simulink model "SimulacionDataRealLaptop"  (R2022b)
settings: Solver=ode4  StartTime=0.0  StopTime=60  FixedStep=0.001  RelTol=1e-3
undefined symbols (not defined in the file): k1, k2, nq, P, W1_0, W2_0
settings Model: Creator=raul  LastModifiedBy=raul

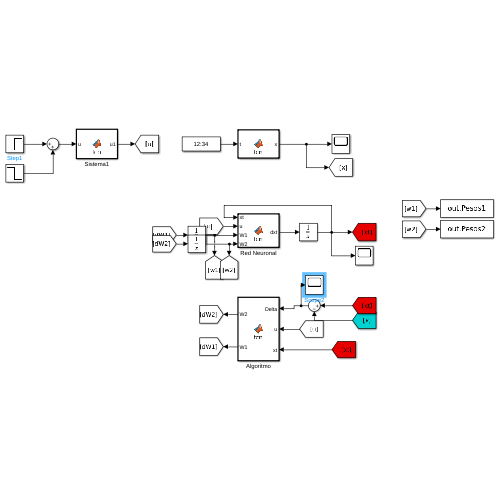
[thumbnail: Simulink's stored preview of the top-level diagram]
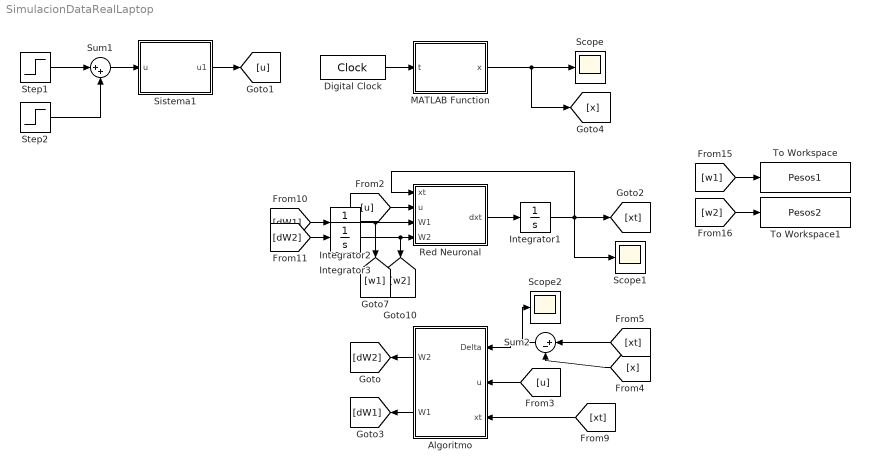
== system SimulacionDataRealLaptop ==
  Algoritmo : MATLAB Function  TreatAsAtomicUnit=on
  Digital Clock : DigitalClock  SampleTime=0.01
  Integrator1 : Integrator  InitialCondition=zeros(2*nq,1)
  Integrator2 : Integrator  InitialCondition=W1_0
  Integrator3 : Integrator  InitialCondition=W2_0
  MATLAB Function : MATLAB Function  TreatAsAtomicUnit=on
  Red Neuronal : MATLAB Function  TreatAsAtomicUnit=on
  Scope : Scope
  Scope1 : Scope
  Scope2 : Scope
  Sistema1 : MATLAB Function  TreatAsAtomicUnit=on
  Step1 : Step  Time=13.50  After=15  SampleTime=0
  Step2 : Step  Time=14  After=-15  SampleTime=0
  Sum1 : Sum  Inputs=|++
  Sum2 : Sum  Inputs=|+-
  To Workspace : ToWorkspace  VariableName=Pesos1  SampleTime=-1
  To Workspace1 : ToWorkspace  VariableName=Pesos2  SampleTime=-1
  wires:
  Digital Clock/1 -> MATLAB Function/1(t)
  MATLAB Function/1(x) -> [x], Scope/1
  [x] -> Sum2/2
  [dW2] -> Integrator3/1
  Integrator3/1 -> [w2], Red Neuronal/4(W2)
  [xt] -> Algoritmo/3(xt)
  Algoritmo/2(W1) -> [dW1]
  Algoritmo/1(W2) -> [dW2]
  [u] -> Algoritmo/2(u)
  [u] -> Red Neuronal/2(u)
  Integrator1/1 -> Scope1/1, [xt], Red Neuronal/1(xt)
  Red Neuronal/1(dxt) -> Integrator1/1
  [xt] -> Sum2/1
  Integrator2/1 -> [w1], Red Neuronal/3(W1)
  [dW1] -> Integrator2/1
  Sum2/1 -> Scope2/1, Algoritmo/1(Delta)
  [w2] -> To Workspace1/1
  [w1] -> To Workspace/1
  Step1/1 -> Sum1/1
  Sum1/1 -> Sistema1/1(u)
  Step2/1 -> Sum1/2
  Sistema1/1(u1) -> [u]

== matlab function SimulacionDataRealLaptop/Algoritmo ==
  data: W2 output; Delta input; P parameter; u input; W1 output; k1 parameter; k2 parameter; xt input
function [W2,W1] = fcn(Delta,P,u, k1, k2,xt)


W1=-k1*P*Delta*sigmoid(1,xt)';
W2=-k2*P*Delta*u'*phi_sigmoid(1,xt)';


function s = sigmoid(b,x)
   s = 1./(1+exp(-b*x)); 
end

function phi=phi_sigmoid(b,xt)
    phi=zeros(20,20);
   for i = 1:20
        for j = 1:20
            phi(i, j) = sigmoid(b, xt(i));
        end
    end
end 

end

== matlab function SimulacionDataRealLaptop/MATLAB Function ==
  data: x output; t input; X parameter
function x = fcn(t, X)

x = X(:,floor(100*t)+1);

== matlab function SimulacionDataRealLaptop/Red Neuronal ==
  data: xt input; u input; dxt output; W1 input; A parameter; W2 input
function dxt = fcn(xt, u, W1, A, W2)

dxt = A*xt+W1*sigmoid(1,xt)+W2*phi_sigmoid(1,xt)*u;


function s = sigmoid(b,x)
   s = 1./(1+exp(-b*x)); 
end

function phi=phi_sigmoid(b,xt)
    phi=zeros(20,20);
   for i = 1:20
        for j = 1:20
            phi(i, j) = sigmoid(b, xt(i));
        end
    end
end 

end

== matlab function SimulacionDataRealLaptop/Sistema1 ==
  data: u1 output; u input
function u1 = fcn(u)%add Bw,w

u1=[0;0;0;0;0;0;0;0;0;u;0;0;0;0;0;0;0;0;0;0];
